simulink model "simulate_data"  (R2022a)
settings: Solver=VariableStepAuto  StartTime=0.0  StopTime=tmax  RelTol=1e-3
values from neighbouring files (symbols this model uses):
  L3 = Y*inv(P)    [lqr_synthesis_observer_simple_Lx3x3_no_VOC.m]
libraries: simulink x1
settings Model: Creator=spinolam  LastModifiedBy=spinolam

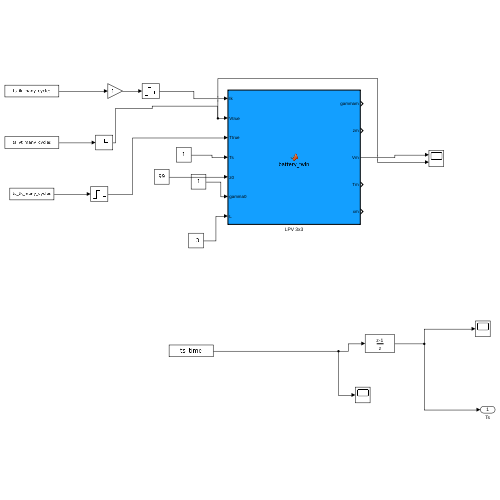
[thumbnail: Simulink's stored preview of the top-level diagram]
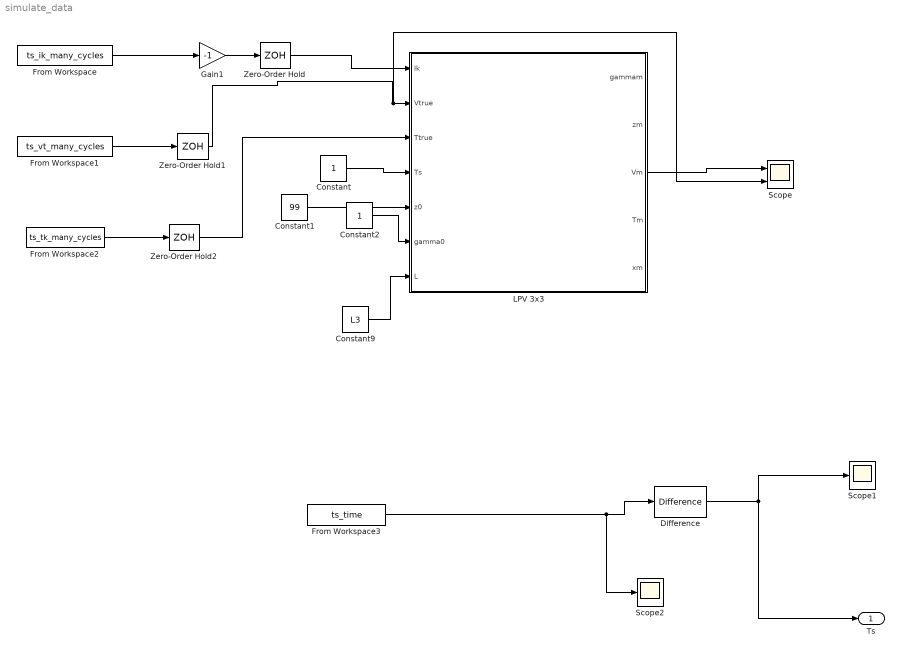
== system simulate_data ==
  Constant : Constant
  Constant1 : Constant  Value=99
  Constant2 : Constant
  Constant9 : Constant  Value=L3  SampleTime=-1
  Difference : simulink/Discrete/Difference  ICPrevInput=0.0  OutMin=[]  OutMax=[]  OutDataType=fixdt(1, 16)  OutScaling=2^-10  DoSatur=off
  From Workspace : FromWorkspace  VariableName=ts_ik_many_cycles  SampleTime=1  Interpolate=off  ZeroCross=off  OutputAfterFinalValue=Setting to zero
  From Workspace1 : FromWorkspace  VariableName=ts_vt_many_cycles  SampleTime=1  Interpolate=off  ZeroCross=off  OutputAfterFinalValue=Setting to zero
  From Workspace2 : FromWorkspace  VariableName=ts_tk_many_cycles  SampleTime=1  Interpolate=off  ZeroCross=off  OutputAfterFinalValue=Setting to zero
  From Workspace3 : FromWorkspace  VariableName=ts_time  OutDataTypeStr=double  SampleTime=1  Interpolate=off  ZeroCross=off  OutputAfterFinalValue=Setting to zero
  Gain1 : Gain  Gain=-1
  LPV 3x3 : MATLAB Function  TreatAsAtomicUnit=on  SystemSampleTime=1
  Scope : Scope  NumInputPorts=2
  Scope1 : Scope
  Scope2 : Scope
  Zero-Order Hold : ZeroOrderHold
  Zero-Order Hold1 : ZeroOrderHold  SampleTime=-1
  Zero-Order Hold2 : ZeroOrderHold  SampleTime=-1
  Ts : Outport
  wires:
  From Workspace/1 -> Gain1/1
  Gain1/1 -> Zero-Order Hold/1
  From Workspace1/1 -> Zero-Order Hold1/1
  From Workspace3/1 -> Difference/1, Scope2/1
  Difference/1 -> Ts/1, Scope1/1
  Zero-Order Hold/1 -> LPV 3x3/1(Ik)
  From Workspace2/1 -> Zero-Order Hold2/1
  Zero-Order Hold2/1 -> LPV 3x3/3(Ttrue)
  Constant/1 -> LPV 3x3/4(Ts)
  Constant1/1 -> LPV 3x3/5(z0)
  Constant2/1 -> LPV 3x3/6(gamma0)
  Constant9/1 -> LPV 3x3/7(L)
  LPV 3x3/3(Vm) -> Scope/1
  Zero-Order Hold1/1 -> Scope/2, LPV 3x3/2(Vtrue)

== matlab function simulate_data/LPV 3x3 ==
  data: Ik input; Vtrue input; Ttrue input; Ts input; gammam output; zm output; Vm output; Tm output; z0 input; gamma0 input; L input; xm output
function [gammam,zm,Vm, Tm,xm]= battery_twin(Ik,Vtrue,Ttrue,Ts, z0, gamma0,L)

persistent zk Vk Tk gammak x Tamb

% params_opt =[0.610556521150227
%    8.598775712524340
%    0.122603898484246
%    2.606767267852760
%    0.192039393270390
%   -0.001348398288203
%    0.000025296007798
%   -0.000000662621556
%    0.000000004414584
%    0.996817945207983
%    2.298831860870833
%   23.000000000000000
% 
% 
% ];
params_opt =[0.919813763352173
   8.599767631518853
   0.273094682411476
   5.142135137038677
   0.094988476730227
  -0.002370241318109
   0.000090365520095
  -0.000001529036050
   0.000000008558929
   0.999025068018285
   8.420763231826188
  23.336063234459374
];
params_opt=[0.919813763352173
   8.599767631518853
   0.273094682411476
   5.142135137038677
   0.094988476730227
  -0.002370241318109
   0.000090365520095
  -0.000001529036050
   0.000000008558929
   0.999025068018285
   8.420763231826188
  23.336063234459374];

params_opt=[0.589068193185747
   8.559272902690564
   0.048189025436034
   3.256250824353102
   0.217261878522855
  -0.000962410714053
   0.000009822495048
  -0.000000423528870
   0.000000002938409
   0.994927725009115
   1.937154456656148
  23.000000000000000];

% --- Parameters Battery ---
N=1;

a=params_opt(1);
% Parameters model Voc
Eo=params_opt(2);
K1=params_opt(3);
K2=params_opt(4);


R0=params_opt(5);
R1=params_opt(6);
R2=params_opt(7);
R3=params_opt(8);
R4=params_opt(9);


%Nominal capacity
Cr =2.5;

% Parameters model temperature
%c2 = 4;
b=params_opt(10); 
c1=params_opt(11);
%Tamb = params_opt(12);
% % --- Parameters Battery ---
% N=1;
% b=0.999; 
% a=0.724851923449880;
% % Parameters model Voc
% Eo=8.455947458036864;
% K1=0.144592227425476;
% K2=0.607377452866854;
% 
% 
% R0=0.216916476498134;
% R1=-0.005249797087054;
% R2=0.000141179901879;
% R3=-0.000002104480344;
% R4=0.000000010785500;
% 
% 
% %Nominal capacity
% Cr =2.5;
% 
% % Parameters model temperature
% %c2 = 4;
% c1=4;
% %Tamb = 23;

% -- Values LPV
%L=[-0.7386   14.3891    0.4483];

%L=0*[-0.270468799102130 0.551733258663858 0.289617027889015];
% N=1;
% b=0.997542721848054; 
% a=0.724851923449880;
% % Parameters model Voc
% Eo=8.455947458036864;
% K1=0.144592227425476;
% K2=0.607377452866854;
% 
% 
% R0=0.216916476498134;
% R1=-0.005249797087054;
% R2=0.000141179901879;
% R3=-0.000002104480344;
% R4=0.000000010785500;
% 
% 
% %Nominal capacity
% Cr =2.5;
% 
% % Parameters model temperature
% %c2 = 4;
% c1=2.310386631071339;
% --- initial states ----
Ik=-Ik;
if isempty(gammak)
    gammak=gamma0;
    
end
if isempty(zk)
    zk=z0;
end
if isempty(Vk) 
    Vk=N*Eo; 
end
if isempty(Tk)
    Tamb=Ttrue; 
    Tk=Tamb; 
end
if isempty(x)
    x=[gamma0;z0;Eo];
end

%L=0*L;
if zk>99.9
    zk=99.9;
end
if zk>99.9
    zk=99.9;
end

% --- map functions -----
Rint=(R0+R1*zk+R2*zk^2+R3*zk^3+R4*zk^4);
Voc=(Eo-K1*log(100-zk)-K2/zk);

% --- dynamic model -----
error=(Vtrue-Vk);
%L=[-0.279587147260702
 %  1.066424440638722
  % 0.267404777088713]';
% --- dynamic model -----
rho1= -100*Ik/(3600*Cr)*Ts;
Rint=N*(R0+R1*x(2)+R2*x(2)^2+R3*x(2)^3+R4*x(2)^4);
rho2= -Ik*Rint;
%Voc=N*(Eo-K1*log(100-x(2))-K2/x(2));
%rho3= Voc/x(2);

L=L;
gamma1 =  1*gammak + L(1)*error;


z1 = zk - Ts*Ik*100*gammak/(3600*Cr)+ L(2)*error;


Ek = Voc-(Rint)*Ik*gammak;
V1 = a*Vk + (1-a)*Ek + L(3)*error;

Tj= Rint*gammak*Ik^2;
T1 = b*Tk + (1-b)*(c1*Tj+Tamb);

A =[ 1 0 0 
       rho1 1 0 
       (1-a)*rho2 0 a ];

B=[0 0 (1-a)*Voc]';
x1 = A*x + B*1+ L*error;

    %sensor model:
zm = zk; % + noise
Vm = Vk; % + noise
gammam =gammak;
Tm=Tk;
xm=x;
%updating z:
x=x1;
zk = z1;
Vk = V1;
Tk=T1;
gammak=gamma1;
